simulink model "standardPcontroller"  (R2020b)
settings: Solver=ode4  StartTime=0.0  StopTime=simulationTime  RelTol=1e-3
undefined symbols (not defined in the file): K, K_p, L, T
settings Model: Creator=Yuto  LastModifiedBy=yuto

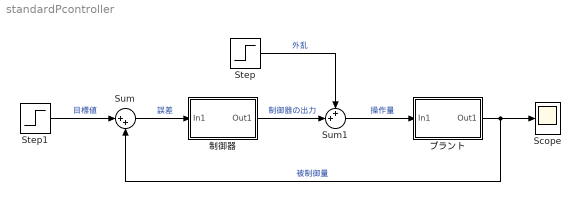
== system standardPcontroller ==
  Scope : Scope
  Step : Step  SampleTime=0
  Step1 : Step  SampleTime=0
  Sum : Sum  Inputs=|++
  Sum1 : Sum  Inputs=++|
  プラント : Subsystem
  制御器 : Subsystem
  wires:
  Step1/1 -> Sum/1  "目標値"
  Step/1 -> Sum1/1  "外乱"
  Sum1/1 -> プラント/1(In1)  "操作量"
  プラント/1(Out1) -> Sum/2, Scope/1  "被制御量"
  Sum/1 -> 制御器/1(In1)  "誤差"
  制御器/1(Out1) -> Sum1/2  "制御器の出力"

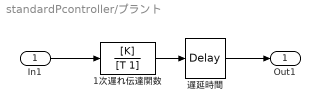
== system standardPcontroller/プラント ==
  In1 : Inport
  1次遅れ伝達関数 : TransferFcn  Numerator=[K]  Denominator=[T 1]
  遅延時間 : TransportDelay  DelayTime=L
  Out1 : Outport
  wires:
  In1/1 -> 1次遅れ伝達関数/1
  1次遅れ伝達関数/1 -> 遅延時間/1
  遅延時間/1 -> Out1/1

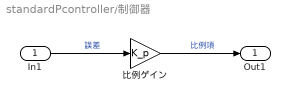
== system standardPcontroller/制御器 ==
  In1 : Inport
  比例ゲイン : Gain  Gain=K_p
  Out1 : Outport
  wires:
  比例ゲイン/1 -> Out1/1  "比例項"
  In1/1 -> 比例ゲイン/1  "誤差"
